simulink model "W07_P1"  (R2024b)
settings: Solver=ode4  StartTime=0  StopTime=T_final  FixedStep=h  RelTol=1e-3
undefined symbols (not defined in the file or in its folder): a_i, beta_c, k_neg, k_pos, k_w, mp, N_slow, phi_i, psi_step, rp, T_max, T_min, T_slow, t_step, V_c, w_i, wave_on, x0, X_ff, y_pont
settings Model: Creator=admin  LastModifiedBy=admin
settings DataIOCC: ReturnWorkspaceOutputs=off

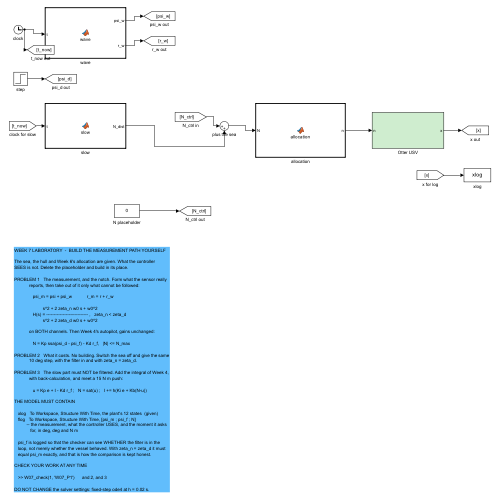
[thumbnail: Simulink's stored preview of the top-level diagram]
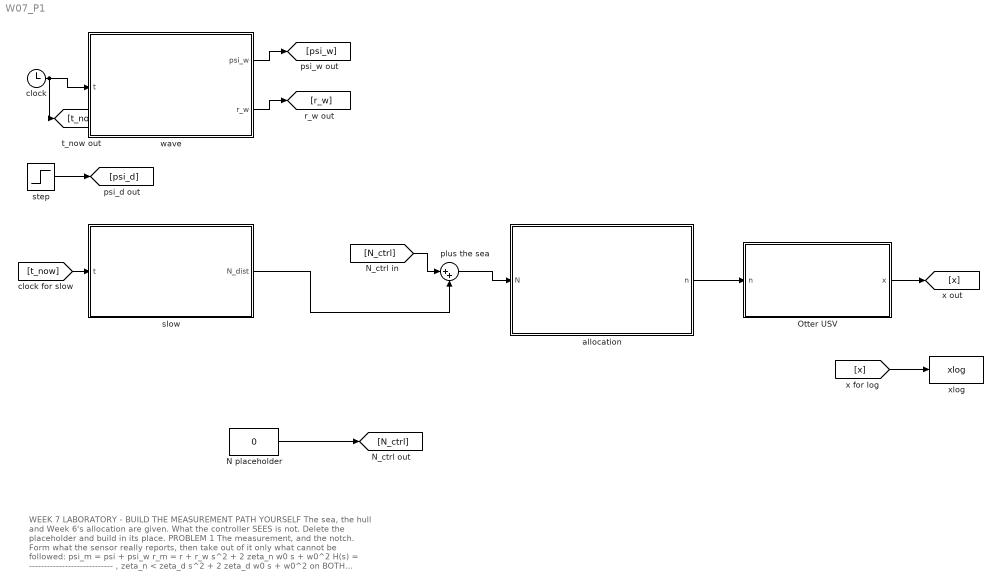
== system W07_P1 ==
  note: WEEK 7 LABORATORY  -  BUILD THE MEASUREMENT PATH YOURSELF
      |
      | The sea, the hull and Week 6's allocation are given. What the controller
      | SEES is not. Delete the placeholder and build in its place.
      |
      | PROBLEM 1   The measurement, and the notch. Form what the sensor really
      |             reports, then take out of it only what cannot be followed:
      |
      |                psi_m = psi + psi_w            r_m = r + r_w
      |
      |                        s^2 + 2 zeta_n w0 s + w0^2
      |                H(s) = ---------------------------- ,   zeta_n < zeta_d
      |                        s^2 + 2 zeta_d w0 s + w0^2
      |
      |             on BOTH channels. Then Week 4's autopilot, gains unchanged:
      |
      |                N = Kp ssa(psi_d - psi_f) - Kd r_f,   |N| <= N_max
      |
      | PROBLEM 2   What it costs. No building. Switch the sea off and give the same
      |             10 deg step, with the filter in and with zeta_n = zeta_d.
      |
      | PROBLEM 3   The slow part must NOT be filtered. Add the integral of Week 4,
      |             with back-calculation, and meet a 15 N m push:
      |
      |                u = Kp e + I - Kd r_f ;   N = sat(u) ;   I += h(Ki e + Kb(N-u))
      |
      | THE MODEL MUST CONTAIN
      |
      |    xlog   To Workspace, Structure With Time, the plant's 12 states  (given)
      |    flog   To Workspace, Structure With Time, [psi_m ; psi_f ; N]
      |           -- the measurement, what the controller USES, and the moment it asks
      |              for, in deg, deg and N m
      |
      |    psi_f is logged so that the checker can see WHETHER the filter is in the
      |    loop, not merely whether the vessel behaved. With zeta_n = zeta_d it must
      |    equal psi_m exactly, and that is how the comparison is kept honest.
      |
      | CHECK YOUR WORK AT ANY TIME
      |
      |    >> W07_check(1, 'W07_P1')      and 2, and 3
      |
      | DO NOT CHANGE the solver settings: fixed-step ode4 at h = 0.02 s.
  N placeholder : Constant  Value=0
  Otter USV : Subsystem
  allocation : MATLAB Function  TreatAsAtomicUnit=on
  clock : Clock
  plus the sea : Sum  Inputs=|++
  slow : MATLAB Function  TreatAsAtomicUnit=on
  step : Step  Time=t_step  After=psi_step  SampleTime=0
  wave : MATLAB Function  TreatAsAtomicUnit=on
  xlog : ToWorkspace  VariableName=xlog  SaveFormat=Structure With Time  SampleTime=-1
  wires:
  clock/1 -> wave/1(t), [t_now]
  wave/1(psi_w) -> [psi_w]
  wave/2(r_w) -> [r_w]
  step/1 -> [psi_d]
  [t_now] -> slow/1(t)
  [N_ctrl] -> plus the sea/1
  slow/1(N_dist) -> plus the sea/2
  plus the sea/1 -> allocation/1(N)
  allocation/1(n) -> Otter USV/1(n)
  Otter USV/1(x) -> [x]
  [x] -> xlog/1
  N placeholder/1 -> [N_ctrl]

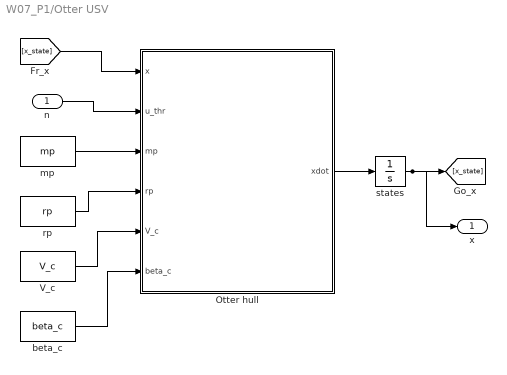
== system W07_P1/Otter USV ==
  n : Inport
  Otter hull : MATLAB Function  TreatAsAtomicUnit=on
  V_c : Constant  Value=V_c
  beta_c : Constant  Value=beta_c
  mp : Constant  Value=mp
  rp : Constant  Value=rp
  states : Integrator  InitialCondition=x0
  x : Outport
  wires:
  [x_state] -> Otter hull/1(x)
  Otter hull/1(xdot) -> states/1
  beta_c/1 -> Otter hull/6(beta_c)
  n/1 -> Otter hull/2(u_thr)
  mp/1 -> Otter hull/3(mp)
  rp/1 -> Otter hull/4(rp)
  V_c/1 -> Otter hull/5(V_c)
  states/1 -> [x_state], x/1

== matlab function W07_P1/slow ==
  data: t input; N_dist output double size=[1 1]; N_slow parameter; T_slow parameter
function N_dist = slow(t, N_slow, T_slow)
%#codegen
%  바람과 2차 파랑 표류를 한 신호로 / wind and second-order drift, as one signal
%
%  파랑(w0 = 3.14 rad/s)보다 두 자리 느리다. 노치는 이것을 **통과시켜야** 한다 —
%  걸러 버리면 제어기가 모르는 사이에 배가 밀려난다.
%  Two decades below the waves. The notch must PASS this: filtered away, the
%  vessel would be pushed off heading without the controller ever seeing it.
N_dist = N_slow*(1 + 0.3*sin(2*pi*t/T_slow));

== matlab function W07_P1/wave ==
  data: t input; psi_w output double size=[1 1]; r_w output; w_i parameter; a_i parameter; phi_i parameter; k_w parameter; wave_on parameter
function [psi_w, r_w] = wave(t, w_i, a_i, phi_i, k_w, wave_on)
%#codegen
%  1차 파랑이 만드는 선수각과 그 변화율 / the wave-induced heading and its rate
%
%      psi_w(t) = k_w sum_i a_i sin(w_i t + phi_i)        [deg]
%      r_w(t)   = k_w sum_i a_i w_i cos(w_i t + phi_i)    [deg/s]
%
%  위상이 정해져 있으므로 이 바다는 매번 똑같다 — 강의의 표를 재현할 수 있다.
%  The phases are fixed, so this sea is the same on every run and the
%  lecture's table can be reproduced.
psi_w = 0;  r_w = 0;
if wave_on ~= 0
    for i = 1:numel(w_i)
        psi_w = psi_w + k_w*a_i(i)*sin(w_i(i)*t + phi_i(i));
        r_w   = r_w   + k_w*a_i(i)*w_i(i)*cos(w_i(i)*t + phi_i(i));
    end
end

== matlab function W07_P1/allocation ==
  data: N input; n output double size=[2 1]; X_ff parameter; y_pont parameter; k_pos parameter; k_neg parameter; T_max parameter; T_min parameter
function n = allocation(N, X_ff, y_pont, k_pos, k_neg, T_max, T_min)
%#codegen
%  6주차의 배분 그대로 / the allocation of Week 6, unchanged
T1 = X_ff/2 + N/(2*y_pont);
T2 = X_ff/2 - N/(2*y_pont);
s = 1;
if T1 > T_max, s = min(s, T_max/T1); end
if T2 > T_max, s = min(s, T_max/T2); end
if T1 < T_min, s = min(s, T_min/T1); end
if T2 < T_min, s = min(s, T_min/T2); end
T1 = s*T1;  T2 = s*T2;
k1 = k_pos;  if T1 < 0, k1 = k_neg; end
k2 = k_pos;  if T2 < 0, k2 = k_neg; end
n = [sign(T1)*sqrt(abs(T1)/k1); sign(T2)*sqrt(abs(T2)/k2)];

== matlab function W07_P1/Otter USV/Otter hull ==
  data: x input; xdot output double size=[12 1]; u_thr input; mp input; rp input; V_c input; beta_c input
function xdot = otter_hull(x, u_thr, mp, rp, V_c, beta_c)
% Fossen's otter.m, called unchanged from Tools/MSS/VESSELS.
%
%   x       12 states, fed back from the integrator
%   u_thr   propeller shaft speeds [rad/s]
%
% otter.m is not written for code generation, so the call is extrinsic and
% xdot has to be pre-sized for Simulink to know the output width.
coder.extrinsic('otter');

xdot = zeros(12,1);
xdot = otter(x, u_thr, mp, rp, V_c, beta_c);
end
